simulink library "inp"  (R2021b)
settings: Solver=VariableStepAuto  StartTime=0.0  StopTime=10.0  RelTol=1e-3
undefined symbols (not defined in the file): C_TASK_5MS_S, FALSE, KINP_AcoreReadyToSlp_flg_ovrdflg, KINP_AcoreReadyToSlp_flg_ovrdval, KINP_AllowMovThd_OTA_enum_ovrdflg, KINP_AllowMovThd_OTA_enum_ovrdval, KINP_APSAngleTarget_Deg_ovrdflg, KINP_APSAngleTarget_Deg_ovrdval, KINP_APSDecReq_mps2_ovrdflg, KINP_APSDecReq_mps2_ovrdval, KINP_APSDecReqA_flg_ovrdflg, KINP_APSDecReqA_flg_ovrdval, KINP_APSDFLL_cm_ovrdflg, KINP_APSDFLL_cm_ovrdval, KINP_APSDFLR_cm_ovrdflg, KINP_APSDFLR_cm_ovrdval, KINP_APSDRLL_cm_ovrdflg, KINP_APSDRLL_cm_ovrdval, KINP_APSDRLR_cm_ovrdflg, KINP_APSDRLR_cm_ovrdval, KINP_APSExitCondition_enum_ovrdflg, KINP_APSExitCondition_enum_ovrdval, KINP_APSHWVer_enum_ovrdflg, KINP_APSHWVer_enum_ovrdval, KINP_APSProgressPCT_pct_ovrdflg, KINP_APSProgressPCT_pct_ovrdval, KINP_APSPwrReq_enum_ovrdflg, KINP_APSPwrReq_enum_ovrdval, KINP_APSReq_enum_ovrdflg, KINP_APSReq_enum_ovrdval, KINP_APSRQDisplay_enum_ovrdflg, KINP_APSRQDisplay_enum_ovrdval, KINP_APSRqEPASCtrl_flg_ovrdflg, KINP_APSRqEPASCtrl_flg_ovrdval, KINP_APSShiftPosnReq_enum_ovrdval, KINP_APSShiftPosnReq_enum_ovrflg, KINP_APSSpeedCMD_kph_ovrdval, KINP_APSSpeedCMD_kph_ovrflg, KINP_APSStaSystem_enum_ovrdflg, KINP_APSStaSystem_enum_ovrdval, KINP_APSSWVer_enum_ovrdflg, KINP_APSSWVer_enum_ovrdval, KINP_APSVMCReqA_flg_ovrdval, KINP_APSVMCReqA_flg_ovrflg, KINP_APSVRqEPASCtrl_flg_ovrdflg, KINP_APSVRqEPASCtrl_flg_ovrdval, KINP_AuxBattVolmV_mV_ovrdflg, KINP_AuxBattVolmV_mV_ovrdval, KINP_CAASSta_enum_ovrdflg, KINP_CAASSta_enum_ovrdval, KINP_CAASVMCReqA_flg_ovrdval, KINP_CAASVMCReqA_flg_ovrflg, KINP_CAN1BusOff_flg_ovrdflg, KINP_CAN1BusOff_flg_ovrdval, KINP_CAN2BusOff_flg_ovrdflg, KINP_CAN2BusOff_flg_ovrdval, KINP_CAN3BusOff_flg_ovrdflg, KINP_CAN3BusOff_flg_ovrdval, KINP_CAN4BusOff_flg_ovrdflg, KINP_CAN4BusOff_flg_ovrdval ... (+152)
libraries: FVT_lib x1037, hcu_lib x1
(part 33 of 34)

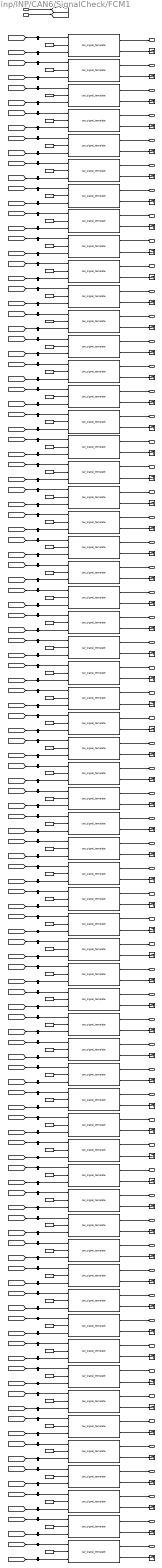
== system inp/INP/CAN6/SignalCheck/FCM1 ==
  BHAL_outputs : Inport
  inp_CanValid_bus : Inport  Port=2
  ACCComfortBandLower : FVT_lib/inp/can_signal_template  SystemSampleTime=-1  VariantActivationTime=update diagram  Latency=0  AutoFrameSizeCalculation=off
      link override defval: Value=KINP_ACCComfortBandLower_mps2_defval
      link override ovrdflg: Value=KINP_ACCComfortBandLower_mps2_ovrdflg
      link override ovrdval: Value=KINP_ACCComfortBandLower_mps2_ovrdval
  ACCComfortBandUpper : FVT_lib/inp/can_signal_template  SystemSampleTime=-1  VariantActivationTime=update diagram  Latency=0  AutoFrameSizeCalculation=off
      link override defval: Value=KINP_ACCComfortBandUpper_mps2_defval
      link override ovrdflg: Value=KINP_ACCComfortBandUpper_mps2_ovrdflg
      link override ovrdval: Value=KINP_ACCComfortBandUpper_mps2_ovrdval
  ACCJerkLowerLimit : FVT_lib/inp/can_signal_template  SystemSampleTime=-1  VariantActivationTime=update diagram  Latency=0  AutoFrameSizeCalculation=off
      link override defval: Value=KINP_ACCJerkLowerLimit_mps3_defval
      link override ovrdflg: Value=KINP_ACCJerkLowerLimit_mps3_ovrdflg
      link override ovrdval: Value=KINP_ACCJerkLowerLimit_mps3_ovrdval
  ACCJerkUpperLimit : FVT_lib/inp/can_signal_template  SystemSampleTime=-1  VariantActivationTime=update diagram  Latency=0  AutoFrameSizeCalculation=off
      link override defval: Value=KINP_ACCJerkUpperLimit_mps3_defval
      link override ovrdflg: Value=KINP_ACCJerkUpperLimit_mps3_ovrdflg
      link override ovrdval: Value=KINP_ACCJerkUpperLimit_mps3_ovrdval
  ACCObjDist : FVT_lib/inp/can_signal_template  SystemSampleTime=-1  VariantActivationTime=update diagram  Latency=0  AutoFrameSizeCalculation=off
      link override defval: Value=KINP_ACCObjDist_m_defval
      link override ovrdflg: Value=KINP_ACCObjDist_m_ovrdflg
      link override ovrdval: Value=KINP_ACCObjDist_m_ovrdval
  ACCObjDstLvl : FVT_lib/inp/can_signal_template  SystemSampleTime=-1  VariantActivationTime=update diagram  Latency=0  AutoFrameSizeCalculation=off
      link override defval: Value=KINP_ACCObjDstLvl_enum_defval
      link override ovrdflg: Value=KINP_ACCObjDstLvl_enum_ovrdflg
      link override ovrdval: Value=KINP_ACCObjDstLvl_enum_ovrdval
  ACCObjRelSpd : FVT_lib/inp/can_signal_template  SystemSampleTime=-1  VariantActivationTime=update diagram  Latency=0  AutoFrameSizeCalculation=off
      link override defval: Value=KINP_ACCObjRelSpd_mps_defval
      link override ovrdflg: Value=KINP_ACCObjRelSpd_mps_ovrdflg
      link override ovrdval: Value=KINP_ACCObjRelSpd_mps_ovrdval
  ACCRequiredAccel : FVT_lib/inp/can_signal_template  SystemSampleTime=-1  VariantActivationTime=update diagram  Latency=0  AutoFrameSizeCalculation=off
      link override defval: Value=KINP_ACCRequiredAccel_mps2_defval
      link override ovrdflg: Value=KINP_ACCRequiredAccel_mps2_ovrdflg
      link override ovrdval: Value=KINP_ACCRequiredAccel_mps2_ovrdval
  ACCTakeoverReq : FVT_lib/inp/can_signal_template  SystemSampleTime=-1  VariantActivationTime=update diagram  Latency=0  AutoFrameSizeCalculation=off
      link override defval: Value=KINP_ACCTakeoverReq_flg_defval
      link override ovrdflg: Value=KINP_ACCTakeoverReq_flg_ovrdflg
      link override ovrdval: Value=KINP_ACCTakeoverReq_flg_ovrdval
  ACCVehHoldReq : FVT_lib/inp/can_signal_template  SystemSampleTime=-1  VariantActivationTime=update diagram  Latency=0  AutoFrameSizeCalculation=off
      link override defval: Value=KINP_ACCVehHoldReq_flg_defval
      link override ovrdflg: Value=KINP_ACCVehHoldReq_flg_ovrdflg
      link override ovrdval: Value=KINP_ACCVehHoldReq_flg_ovrdval
  ADASACCSta : FVT_lib/inp/can_signal_template  SystemSampleTime=-1  VariantActivationTime=update diagram  Latency=0  AutoFrameSizeCalculation=off
      link override defval: Value=KINP_ADASACCSta_enum_defval
      link override ovrdflg: Value=KINP_ADASACCSta_enum_ovrdflg
      link override ovrdval: Value=KINP_ADASACCSta_enum_ovrdval
  ADASAEBReq : FVT_lib/inp/can_signal_template  SystemSampleTime=-1  VariantActivationTime=update diagram  Latency=0  AutoFrameSizeCalculation=off
      link override defval: Value=KINP_ADASAEBReq_enum_defval
      link override ovrdflg: Value=KINP_ADASAEBReq_enum_ovrdflg
      link override ovrdval: Value=KINP_ADASAEBReq_enum_ovrdval
  ADASAEBSta : FVT_lib/inp/can_signal_template  SystemSampleTime=-1  VariantActivationTime=update diagram  Latency=0  AutoFrameSizeCalculation=off
      link override defval: Value=KINP_ADASAEBSta_enum_defval
      link override ovrdflg: Value=KINP_ADASAEBSta_enum_ovrdflg
      link override ovrdval: Value=KINP_ADASAEBSta_enum_ovrdval
  ADASCAMSpdLim : FVT_lib/inp/can_signal_template  SystemSampleTime=-1  VariantActivationTime=update diagram  Latency=0  AutoFrameSizeCalculation=off
      link override defval: Value=KINP_ADASCAMSpdLim_enum_defval
      link override ovrdflg: Value=KINP_ADASCAMSpdLim_enum_ovrdflg
      link override ovrdval: Value=KINP_ADASCAMSpdLim_enum_ovrdval
  ADASDBSReq : FVT_lib/inp/can_signal_template  SystemSampleTime=-1  VariantActivationTime=update diagram  Latency=0  AutoFrameSizeCalculation=off
      link override defval: Value=KINP_ADASDBSReq_enum_defval
      link override ovrdflg: Value=KINP_ADASDBSReq_enum_ovrdflg
      link override ovrdval: Value=KINP_ADASDBSReq_enum_ovrdval
  ADASFCWMute : FVT_lib/inp/can_signal_template  SystemSampleTime=-1  VariantActivationTime=update diagram  Latency=0  AutoFrameSizeCalculation=off
      link override defval: Value=KINP_ADASFCWMute_flg_defval
      link override ovrdflg: Value=KINP_ADASFCWMute_flg_ovrdflg
      link override ovrdval: Value=KINP_ADASFCWMute_flg_ovrdval
  ADASFCWSta : FVT_lib/inp/can_signal_template  SystemSampleTime=-1  VariantActivationTime=update diagram  Latency=0  AutoFrameSizeCalculation=off
      link override defval: Value=KINP_ADASFCWSta_enum_defval
      link override ovrdflg: Value=KINP_ADASFCWSta_enum_ovrdflg
      link override ovrdval: Value=KINP_ADASFCWSta_enum_ovrdval
  ADASFaultSta : FVT_lib/inp/can_signal_template  SystemSampleTime=-1  VariantActivationTime=update diagram  Latency=0  AutoFrameSizeCalculation=off
      link override defval: Value=KINP_ADASFaultSta_flg_defval
      link override ovrdflg: Value=KINP_ADASFaultSta_flg_ovrdflg
      link override ovrdval: Value=KINP_ADASFaultSta_flg_ovrdval
  ADASFltWrnReq : FVT_lib/inp/can_signal_template  SystemSampleTime=-1  VariantActivationTime=update diagram  Latency=0  AutoFrameSizeCalculation=off
      link override defval: Value=KINP_ADASFltWrnReq_flg_defval
      link override ovrdflg: Value=KINP_ADASFltWrnReq_flg_ovrdflg
      link override ovrdval: Value=KINP_ADASFltWrnReq_flg_ovrdval
  ADASForceIdle : FVT_lib/inp/can_signal_template  SystemSampleTime=-1  VariantActivationTime=update diagram  Latency=0  AutoFrameSizeCalculation=off
      link override defval: Value=KINP_ADASForceIdle_flg_defval
      link override ovrdflg: Value=KINP_ADASForceIdle_flg_ovrdflg
      link override ovrdval: Value=KINP_ADASForceIdle_flg_ovrdval
  ADASISASta : FVT_lib/inp/can_signal_template  SystemSampleTime=-1  VariantActivationTime=update diagram  Latency=0  AutoFrameSizeCalculation=off
      link override defval: Value=KINP_ADASISASta_enum_defval
      link override ovrdflg: Value=KINP_ADASISASta_enum_ovrdflg
      link override ovrdval: Value=KINP_ADASISASta_enum_ovrdval
  ADASLDWMute : FVT_lib/inp/can_signal_template  SystemSampleTime=-1  VariantActivationTime=update diagram  Latency=0  AutoFrameSizeCalculation=off
      link override defval: Value=KINP_ADASLDWMute_flg_defval
      link override ovrdflg: Value=KINP_ADASLDWMute_flg_ovrdflg
      link override ovrdval: Value=KINP_ADASLDWMute_flg_ovrdval
  ADASLDWSta : FVT_lib/inp/can_signal_template  SystemSampleTime=-1  VariantActivationTime=update diagram  Latency=0  AutoFrameSizeCalculation=off
      link override defval: Value=KINP_ADASLDWSta_enum_defval
      link override ovrdflg: Value=KINP_ADASLDWSta_enum_ovrdflg
      link override ovrdval: Value=KINP_ADASLDWSta_enum_ovrdval
  ADASLFCHandsOffWarning : FVT_lib/inp/can_signal_template  SystemSampleTime=-1  VariantActivationTime=update diagram  Latency=0  AutoFrameSizeCalculation=off
      link override defval: Value=KINP_ADASLFCHandsOffWarning_enum_defval
      link override ovrdflg: Value=KINP_ADASLFCHandsOffWarning_enum_ovrdflg
      link override ovrdval: Value=KINP_ADASLFCHandsOffWarning_enum_ovrdval
  ADASLFCSta : FVT_lib/inp/can_signal_template  SystemSampleTime=-1  VariantActivationTime=update diagram  Latency=0  AutoFrameSizeCalculation=off
      link override defval: Value=KINP_ADASLFCSta_enum_defval
      link override ovrdflg: Value=KINP_ADASLFCSta_enum_ovrdflg
      link override ovrdval: Value=KINP_ADASLFCSta_enum_ovrdval
  ADASLFCWarnSound : FVT_lib/inp/can_signal_template  SystemSampleTime=-1  VariantActivationTime=update diagram  Latency=0  AutoFrameSizeCalculation=off
      link override defval: Value=KINP_ADASLFCWarnSound_enum_defval
      link override ovrdflg: Value=KINP_ADASLFCWarnSound_enum_ovrdflg
      link override ovrdval: Value=KINP_ADASLFCWarnSound_enum_ovrdval
  ADASLKASta : FVT_lib/inp/can_signal_template  SystemSampleTime=-1  VariantActivationTime=update diagram  Latency=0  AutoFrameSizeCalculation=off
      link override defval: Value=KINP_ADASLKASta_enum_defval
      link override ovrdflg: Value=KINP_ADASLKASta_enum_ovrdflg
      link override ovrdval: Value=KINP_ADASLKASta_enum_ovrdval
  ADASLaneModeL : FVT_lib/inp/can_signal_template  SystemSampleTime=-1  VariantActivationTime=update diagram  Latency=0  AutoFrameSizeCalculation=off
      link override defval: Value=KINP_ADASLaneModeL_enum_defval
      link override ovrdflg: Value=KINP_ADASLaneModeL_enum_ovrdflg
      link override ovrdval: Value=KINP_ADASLaneModeL_enum_ovrdval
  ADASLaneModeR : FVT_lib/inp/can_signal_template  SystemSampleTime=-1  VariantActivationTime=update diagram  Latency=0  AutoFrameSizeCalculation=off
      link override defval: Value=KINP_ADASLaneModeR_enum_defval
      link override ovrdflg: Value=KINP_ADASLaneModeR_enum_ovrdflg
      link override ovrdval: Value=KINP_ADASLaneModeR_enum_ovrdval
  ADASLanecurveL : FVT_lib/inp/can_signal_template  SystemSampleTime=-1  VariantActivationTime=update diagram  Latency=0  AutoFrameSizeCalculation=off
      link override defval: Value=KINP_ADASLanecurveL_raw32_defval
      link override ovrdflg: Value=KINP_ADASLanecurveL_raw32_ovrdflg
      link override ovrdval: Value=KINP_ADASLanecurveL_raw32_ovrdval
  ADASLanecurveR : FVT_lib/inp/can_signal_template  SystemSampleTime=-1  VariantActivationTime=update diagram  Latency=0  AutoFrameSizeCalculation=off
      link override defval: Value=KINP_ADASLanecurveR_raw32_defval
      link override ovrdflg: Value=KINP_ADASLanecurveR_raw32_ovrdflg
      link override ovrdval: Value=KINP_ADASLanecurveR_raw32_ovrdval
  ADASLanetypeL : FVT_lib/inp/can_signal_template  SystemSampleTime=-1  VariantActivationTime=update diagram  Latency=0  AutoFrameSizeCalculation=off
      link override defval: Value=KINP_ADASLanetypeL_enum_defval
      link override ovrdflg: Value=KINP_ADASLanetypeL_enum_ovrdflg
      link override ovrdval: Value=KINP_ADASLanetypeL_enum_ovrdval
  ADASLanetypeR : FVT_lib/inp/can_signal_template  SystemSampleTime=-1  VariantActivationTime=update diagram  Latency=0  AutoFrameSizeCalculation=off
      link override defval: Value=KINP_ADASLanetypeR_enum_defval
      link override ovrdflg: Value=KINP_ADASLanetypeR_enum_ovrdflg
      link override ovrdval: Value=KINP_ADASLanetypeR_enum_ovrdval
  ADASSLIFSpdLim : FVT_lib/inp/can_signal_template  SystemSampleTime=-1  VariantActivationTime=update diagram  Latency=0  AutoFrameSizeCalculation=off
      link override defval: Value=KINP_ADASSLIFSpdLim_enum_defval
      link override ovrdflg: Value=KINP_ADASSLIFSpdLim_enum_ovrdflg
      link override ovrdval: Value=KINP_ADASSLIFSpdLim_enum_ovrdval
  ADASSLIFSta : FVT_lib/inp/can_signal_template  SystemSampleTime=-1  VariantActivationTime=update diagram  Latency=0  AutoFrameSizeCalculation=off
      link override defval: Value=KINP_ADASSLIFSta_enum_defval
      link override ovrdflg: Value=KINP_ADASSLIFSta_enum_ovrdflg
      link override ovrdval: Value=KINP_ADASSLIFSta_enum_ovrdval
  ADASShftPosnReq : FVT_lib/inp/can_signal_template  SystemSampleTime=-1  VariantActivationTime=update diagram  Latency=0  AutoFrameSizeCalculation=off
      link override defval: Value=KINP_ADASShftPosnReq_enum_defval
      link override ovrdflg: Value=KINP_ADASShftPosnReq_enum_ovrdflg
      link override ovrdval: Value=KINP_ADASShftPosnReq_enum_ovrdval
  ADASShftPosnReqA : FVT_lib/inp/can_signal_template  SystemSampleTime=-1  VariantActivationTime=update diagram  Latency=0  AutoFrameSizeCalculation=off
      link override defval: Value=KINP_ADASShftPosnReqA_flg_defval
      link override ovrdflg: Value=KINP_ADASShftPosnReqA_flg_ovrdflg
      link override ovrdval: Value=KINP_ADASShftPosnReqA_flg_ovrdval
  ADASVehSpdLim : FVT_lib/inp/can_signal_template  SystemSampleTime=-1  VariantActivationTime=update diagram  Latency=0  AutoFrameSizeCalculation=off
      link override defval: Value=KINP_ADASVehSpdLim_enum_defval
      link override ovrdflg: Value=KINP_ADASVehSpdLim_enum_ovrdflg
      link override ovrdval: Value=KINP_ADASVehSpdLim_enum_ovrdval
  ADASWarningMsg : FVT_lib/inp/can_signal_template  SystemSampleTime=-1  VariantActivationTime=update diagram  Latency=0  AutoFrameSizeCalculation=off
      link override defval: Value=KINP_ADASWarningMsg_enum_defval
      link override ovrdflg: Value=KINP_ADASWarningMsg_enum_ovrdflg
      link override ovrdval: Value=KINP_ADASWarningMsg_enum_ovrdval
  AEBVehHoldReq : FVT_lib/inp/can_signal_template  SystemSampleTime=-1  VariantActivationTime=update diagram  Latency=0  AutoFrameSizeCalculation=off
      link override defval: Value=KINP_AEBVehHoldReq_flg_defval
      link override ovrdflg: Value=KINP_AEBVehHoldReq_flg_ovrdflg
      link override ovrdval: Value=KINP_AEBVehHoldReq_flg_ovrdval
  CameraBlockage : FVT_lib/inp/can_signal_template  SystemSampleTime=-1  VariantActivationTime=update diagram  Latency=0  AutoFrameSizeCalculation=off
      link override defval: Value=KINP_CameraBlockage_flg_defval
      link override ovrdflg: Value=KINP_CameraBlockage_flg_ovrdflg
      link override ovrdval: Value=KINP_CameraBlockage_flg_ovrdval
  FCM1Checksum : FVT_lib/inp/can_signal_template  SystemSampleTime=-1  VariantActivationTime=update diagram  Latency=0  AutoFrameSizeCalculation=off
      link override defval: Value=KINP_FCM1Checksum_enum_defval
      link override ovrdflg: Value=KINP_FCM1Checksum_enum_ovrdflg
      link override ovrdval: Value=KINP_FCM1Checksum_enum_ovrdval
  FCM1LifeCount : FVT_lib/inp/can_signal_template  SystemSampleTime=-1  VariantActivationTime=update diagram  Latency=0  AutoFrameSizeCalculation=off
      link override defval: Value=KINP_FCM1LifeCount_enum_defval
      link override ovrdflg: Value=KINP_FCM1LifeCount_enum_ovrdflg
      link override ovrdval: Value=KINP_FCM1LifeCount_enum_ovrdval
  FCMACCmode : FVT_lib/inp/can_signal_template  SystemSampleTime=-1  VariantActivationTime=update diagram  Latency=0  AutoFrameSizeCalculation=off
      link override defval: Value=KINP_FCMACCmode_enum_defval
      link override ovrdflg: Value=KINP_FCMACCmode_enum_ovrdflg
      link override ovrdval: Value=KINP_FCMACCmode_enum_ovrdval
  FCMLKAStrToqReq : FVT_lib/inp/can_signal_template  SystemSampleTime=-1  VariantActivationTime=update diagram  Latency=0  AutoFrameSizeCalculation=off
      link override defval: Value=KINP_FCMLKAStrToqReq_Nm_defval
      link override ovrdflg: Value=KINP_FCMLKAStrToqReq_Nm_ovrdflg
      link override ovrdval: Value=KINP_FCMLKAStrToqReq_Nm_ovrdval
  FCMLKATOIAct : FVT_lib/inp/can_signal_template  SystemSampleTime=-1  VariantActivationTime=update diagram  Latency=0  AutoFrameSizeCalculation=off
      link override defval: Value=KINP_FCMLKATOIAct_enum_defval
      link override ovrdflg: Value=KINP_FCMLKATOIAct_enum_ovrdflg
      link override ovrdval: Value=KINP_FCMLKATOIAct_enum_ovrdval
  FCMLKATOIFault : FVT_lib/inp/can_signal_template  SystemSampleTime=-1  VariantActivationTime=update diagram  Latency=0  AutoFrameSizeCalculation=off
      link override defval: Value=KINP_FCMLKATOIFault_flg_defval
      link override ovrdflg: Value=KINP_FCMLKATOIFault_flg_ovrdflg
      link override ovrdval: Value=KINP_FCMLKATOIFault_flg_ovrdval
  ForceLowBeam : FVT_lib/inp/can_signal_template  SystemSampleTime=-1  VariantActivationTime=update diagram  Latency=0  AutoFrameSizeCalculation=off
      link override defval: Value=KINP_ForceLowBeam_enum_defval
      link override ovrdflg: Value=KINP_ForceLowBeam_enum_ovrdflg
      link override ovrdval: Value=KINP_ForceLowBeam_enum_ovrdval
  HazardWarningReq : FVT_lib/inp/can_signal_template  SystemSampleTime=-1  VariantActivationTime=update diagram  Latency=0  AutoFrameSizeCalculation=off
      link override defval: Value=KINP_HazardWarningReq_flg_defval
      link override ovrdflg: Value=KINP_HazardWarningReq_flg_ovrdflg
      link override ovrdval: Value=KINP_HazardWarningReq_flg_ovrdval
  ISAWarningMsg : FVT_lib/inp/can_signal_template  SystemSampleTime=-1  VariantActivationTime=update diagram  Latency=0  AutoFrameSizeCalculation=off
      link override defval: Value=KINP_ISAWarningMsg_enum_defval
      link override ovrdflg: Value=KINP_ISAWarningMsg_enum_ovrdflg
      link override ovrdval: Value=KINP_ISAWarningMsg_enum_ovrdval
  LKAHODDisplayWarning : FVT_lib/inp/can_signal_template  SystemSampleTime=-1  VariantActivationTime=update diagram  Latency=0  AutoFrameSizeCalculation=off
      link override defval: Value=KINP_LKAHODDisplayWarning_flg_defval
      link override ovrdflg: Value=KINP_LKAHODDisplayWarning_flg_ovrdflg
      link override ovrdval: Value=KINP_LKAHODDisplayWarning_flg_ovrdval
  LKAHODSoundWarning : FVT_lib/inp/can_signal_template  SystemSampleTime=-1  VariantActivationTime=update diagram  Latency=0  AutoFrameSizeCalculation=off
      link override defval: Value=KINP_LKAHODSoundWarning_flg_defval
      link override ovrdflg: Value=KINP_LKAHODSoundWarning_flg_ovrdflg
      link override ovrdval: Value=KINP_LKAHODSoundWarning_flg_ovrdval
  LVDAACCStatusInformation : FVT_lib/inp/can_signal_template  SystemSampleTime=-1  VariantActivationTime=update diagram  Latency=0  AutoFrameSizeCalculation=off
      link override defval: Value=KINP_LVDAACCStatusInformation_flg_defval
      link override ovrdflg: Value=KINP_LVDAACCStatusInformation_flg_ovrdflg
      link override ovrdval: Value=KINP_LVDAACCStatusInformation_flg_ovrdval
  LVDADisabled : FVT_lib/inp/can_signal_template  SystemSampleTime=-1  VariantActivationTime=update diagram  Latency=0  AutoFrameSizeCalculation=off
      link override defval: Value=KINP_LVDADisabled_flg_defval
      link override ovrdflg: Value=KINP_LVDADisabled_flg_ovrdflg
      link override ovrdval: Value=KINP_LVDADisabled_flg_ovrdval
  LVDAFailinfo : FVT_lib/inp/can_signal_template  SystemSampleTime=-1  VariantActivationTime=update diagram  Latency=0  AutoFrameSizeCalculation=off
      link override defval: Value=KINP_LVDAFailinfo_flg_defval
      link override ovrdflg: Value=KINP_LVDAFailinfo_flg_ovrdflg
      link override ovrdval: Value=KINP_LVDAFailinfo_flg_ovrdval
  LVDAMuteSta : FVT_lib/inp/can_signal_template  SystemSampleTime=-1  VariantActivationTime=update diagram  Latency=0  AutoFrameSizeCalculation=off
      link override defval: Value=KINP_LVDAMuteSta_enum_defval
      link override ovrdflg: Value=KINP_LVDAMuteSta_enum_ovrdflg
      link override ovrdval: Value=KINP_LVDAMuteSta_enum_ovrdval
  LVDAWarning : FVT_lib/inp/can_signal_template  SystemSampleTime=-1  VariantActivationTime=update diagram  Latency=0  AutoFrameSizeCalculation=off
      link override defval: Value=KINP_LVDAWarning_flg_defval
      link override ovrdflg: Value=KINP_LVDAWarning_flg_ovrdflg
      link override ovrdval: Value=KINP_LVDAWarning_flg_ovrdval
  LeftTurnLightReq : FVT_lib/inp/can_signal_template  SystemSampleTime=-1  VariantActivationTime=update diagram  Latency=0  AutoFrameSizeCalculation=off
      link override defval: Value=KINP_LeftTurnLightReq_flg_defval
      link override ovrdflg: Value=KINP_LeftTurnLightReq_flg_ovrdflg
      link override ovrdval: Value=KINP_LeftTurnLightReq_flg_ovrdval
  RightTurnLightReq : FVT_lib/inp/can_signal_template  SystemSampleTime=-1  VariantActivationTime=update diagram  Latency=0  AutoFrameSizeCalculation=off
      link override defval: Value=KINP_RightTurnLightReq_flg_defval
      link override ovrdflg: Value=KINP_RightTurnLightReq_flg_ovrdflg
      link override ovrdval: Value=KINP_RightTurnLightReq_flg_ovrdval
  TargetType : FVT_lib/inp/can_signal_template  SystemSampleTime=-1  VariantActivationTime=update diagram  Latency=0  AutoFrameSizeCalculation=off
      link override defval: Value=KINP_TargetType_enum_defval
      link override ovrdflg: Value=KINP_TargetType_enum_ovrdflg
      link override ovrdval: Value=KINP_TargetType_enum_ovrdval
  Terminator_{1..61} (61 alike) : Terminator
  TimeGapLevel : FVT_lib/inp/can_signal_template  SystemSampleTime=-1  VariantActivationTime=update diagram  Latency=0  AutoFrameSizeCalculation=off
      link override defval: Value=KINP_TimeGapLevel_enum_defval
      link override ovrdflg: Value=KINP_TimeGapLevel_enum_ovrdflg
      link override ovrdval: Value=KINP_TimeGapLevel_enum_ovrdval
  True_VHAL_ACCComfortBandLower_mps2 : Constant  Value=TRUE  OutDataTypeStr=boolean
  True_VHAL_ACCComfortBandUpper_mps2 : Constant  Value=TRUE  OutDataTypeStr=boolean
  True_VHAL_ACCJerkLowerLimit_mps3 : Constant  Value=TRUE  OutDataTypeStr=boolean
  True_VHAL_ACCJerkUpperLimit_mps3 : Constant  Value=TRUE  OutDataTypeStr=boolean
  True_VHAL_ACCObjDist_m : Constant  Value=TRUE  OutDataTypeStr=boolean
  True_VHAL_ACCObjDstLvl_enum : Constant  Value=TRUE  OutDataTypeStr=boolean
  True_VHAL_ACCObjRelSpd_mps : Constant  Value=TRUE  OutDataTypeStr=boolean
  True_VHAL_ACCRequiredAccel_mps2 : Constant  Value=TRUE  OutDataTypeStr=boolean
  True_VHAL_ACCTakeoverReq_flg : Constant  Value=TRUE  OutDataTypeStr=boolean
  True_VHAL_ACCVehHoldReq_flg : Constant  Value=TRUE  OutDataTypeStr=boolean
  True_VHAL_ADASACCSta_enum : Constant  Value=TRUE  OutDataTypeStr=boolean
  True_VHAL_ADASAEBReq_enum : Constant  Value=TRUE  OutDataTypeStr=boolean
  True_VHAL_ADASAEBSta_enum : Constant  Value=TRUE  OutDataTypeStr=boolean
  True_VHAL_ADASCAMSpdLim_enum : Constant  Value=TRUE  OutDataTypeStr=boolean
  True_VHAL_ADASDBSReq_enum : Constant  Value=TRUE  OutDataTypeStr=boolean
  True_VHAL_ADASFCWMute_flg : Constant  Value=TRUE  OutDataTypeStr=boolean
  True_VHAL_ADASFCWSta_enum : Constant  Value=TRUE  OutDataTypeStr=boolean
  True_VHAL_ADASFaultSta_flg : Constant  Value=TRUE  OutDataTypeStr=boolean
  True_VHAL_ADASFltWrnReq_flg : Constant  Value=TRUE  OutDataTypeStr=boolean
  True_VHAL_ADASForceIdle_flg : Constant  Value=TRUE  OutDataTypeStr=boolean
  True_VHAL_ADASISASta_enum : Constant  Value=TRUE  OutDataTypeStr=boolean
  True_VHAL_ADASLDWMute_flg : Constant  Value=TRUE  OutDataTypeStr=boolean
  True_VHAL_ADASLDWSta_enum : Constant  Value=TRUE  OutDataTypeStr=boolean
  True_VHAL_ADASLFCHandsOffWarning_enum : Constant  Value=TRUE  OutDataTypeStr=boolean
  True_VHAL_ADASLFCSta_enum : Constant  Value=TRUE  OutDataTypeStr=boolean
  True_VHAL_ADASLFCWarnSound_enum : Constant  Value=TRUE  OutDataTypeStr=boolean
  True_VHAL_ADASLKASta_enum : Constant  Value=TRUE  OutDataTypeStr=boolean
  True_VHAL_ADASLaneModeL_enum : Constant  Value=TRUE  OutDataTypeStr=boolean
  True_VHAL_ADASLaneModeR_enum : Constant  Value=TRUE  OutDataTypeStr=boolean
  True_VHAL_ADASLanecurveL_raw32 : Constant  Value=TRUE  OutDataTypeStr=boolean
  True_VHAL_ADASLanecurveR_raw32 : Constant  Value=TRUE  OutDataTypeStr=boolean
  True_VHAL_ADASLanetypeL_enum : Constant  Value=TRUE  OutDataTypeStr=boolean
  True_VHAL_ADASLanetypeR_enum : Constant  Value=TRUE  OutDataTypeStr=boolean
  True_VHAL_ADASSLIFSpdLim_enum : Constant  Value=TRUE  OutDataTypeStr=boolean
  True_VHAL_ADASSLIFSta_enum : Constant  Value=TRUE  OutDataTypeStr=boolean
  True_VHAL_ADASShftPosnReqA_flg : Constant  Value=TRUE  OutDataTypeStr=boolean
  True_VHAL_ADASShftPosnReq_enum : Constant  Value=TRUE  OutDataTypeStr=boolean
  True_VHAL_ADASVehSpdLim_enum : Constant  Value=TRUE  OutDataTypeStr=boolean
  True_VHAL_ADASWarningMsg_enum : Constant  Value=TRUE  OutDataTypeStr=boolean
  True_VHAL_AEBVehHoldReq_flg : Constant  Value=TRUE  OutDataTypeStr=boolean
  True_VHAL_CameraBlockage_flg : Constant  Value=TRUE  OutDataTypeStr=boolean
  True_VHAL_FCM1Checksum_enum : Constant  Value=TRUE  OutDataTypeStr=boolean
  True_VHAL_FCM1LifeCount_enum : Constant  Value=TRUE  OutDataTypeStr=boolean
  True_VHAL_FCMACCmode_enum : Constant  Value=TRUE  OutDataTypeStr=boolean
  True_VHAL_FCMLKAStrToqReq_Nm : Constant  Value=TRUE  OutDataTypeStr=boolean
  True_VHAL_FCMLKATOIAct_enum : Constant  Value=TRUE  OutDataTypeStr=boolean
  True_VHAL_FCMLKATOIFault_flg : Constant  Value=TRUE  OutDataTypeStr=boolean
  True_VHAL_ForceLowBeam_enum : Constant  Value=TRUE  OutDataTypeStr=boolean
  True_VHAL_HazardWarningReq_flg : Constant  Value=TRUE  OutDataTypeStr=boolean
  True_VHAL_ISAWarningMsg_enum : Constant  Value=TRUE  OutDataTypeStr=boolean
  True_VHAL_LKAHODDisplayWarning_flg : Constant  Value=TRUE  OutDataTypeStr=boolean
  True_VHAL_LKAHODSoundWarning_flg : Constant  Value=TRUE  OutDataTypeStr=boolean
  True_VHAL_LVDAACCStatusInformation_flg : Constant  Value=TRUE  OutDataTypeStr=boolean
  True_VHAL_LVDADisabled_flg : Constant  Value=TRUE  OutDataTypeStr=boolean
  True_VHAL_LVDAFailinfo_flg : Constant  Value=TRUE  OutDataTypeStr=boolean
  True_VHAL_LVDAMuteSta_enum : Constant  Value=TRUE  OutDataTypeStr=boolean
  True_VHAL_LVDAWarning_flg : Constant  Value=TRUE  OutDataTypeStr=boolean
  True_VHAL_LeftTurnLightReq_flg : Constant  Value=TRUE  OutDataTypeStr=boolean
  True_VHAL_RightTurnLightReq_flg : Constant  Value=TRUE  OutDataTypeStr=boolean
  True_VHAL_TargetType_enum : Constant  Value=TRUE  OutDataTypeStr=boolean
  True_VHAL_TimeGapLevel_enum : Constant  Value=TRUE  OutDataTypeStr=boolean
  slr1_{1..61} (61 alike) : BusSelector  OutputSignals=VINP_CANMsgValidFCM1_flg
  slr_VHAL_ACCComfortBandLower_mps2 : BusSelector  OutputSignals=VHAL_ACCComfortBandLower_mps2
  slr_VHAL_ACCComfortBandUpper_mps2 : BusSelector  OutputSignals=VHAL_ACCComfortBandUpper_mps2
  slr_VHAL_ACCJerkLowerLimit_mps3 : BusSelector  OutputSignals=VHAL_ACCJerkLowerLimit_mps3
  slr_VHAL_ACCJerkUpperLimit_mps3 : BusSelector  OutputSignals=VHAL_ACCJerkUpperLimit_mps3
  slr_VHAL_ACCObjDist_m : BusSelector  OutputSignals=VHAL_ACCObjDist_m
  slr_VHAL_ACCObjDstLvl_enum : BusSelector  OutputSignals=VHAL_ACCObjDstLvl_enum
  slr_VHAL_ACCObjRelSpd_mps : BusSelector  OutputSignals=VHAL_ACCObjRelSpd_mps
  slr_VHAL_ACCRequiredAccel_mps2 : BusSelector  OutputSignals=VHAL_ACCRequiredAccel_mps2
  slr_VHAL_ACCTakeoverReq_flg : BusSelector  OutputSignals=VHAL_ACCTakeoverReq_flg
  slr_VHAL_ACCVehHoldReq_flg : BusSelector  OutputSignals=VHAL_ACCVehHoldReq_flg
  slr_VHAL_ADASACCSta_enum : BusSelector  OutputSignals=VHAL_ADASACCSta_enum
  slr_VHAL_ADASAEBReq_enum : BusSelector  OutputSignals=VHAL_ADASAEBReq_enum
  slr_VHAL_ADASAEBSta_enum : BusSelector  OutputSignals=VHAL_ADASAEBSta_enum
  slr_VHAL_ADASCAMSpdLim_enum : BusSelector  OutputSignals=VHAL_ADASCAMSpdLim_enum
  slr_VHAL_ADASDBSReq_enum : BusSelector  OutputSignals=VHAL_ADASDBSReq_enum
  slr_VHAL_ADASFCWMute_flg : BusSelector  OutputSignals=VHAL_ADASFCWMute_flg
  slr_VHAL_ADASFCWSta_enum : BusSelector  OutputSignals=VHAL_ADASFCWSta_enum
  slr_VHAL_ADASFaultSta_flg : BusSelector  OutputSignals=VHAL_ADASFaultSta_flg
  slr_VHAL_ADASFltWrnReq_flg : BusSelector  OutputSignals=VHAL_ADASFltWrnReq_flg
  slr_VHAL_ADASForceIdle_flg : BusSelector  OutputSignals=VHAL_ADASForceIdle_flg
  slr_VHAL_ADASISASta_enum : BusSelector  OutputSignals=VHAL_ADASISASta_enum
  slr_VHAL_ADASLDWMute_flg : BusSelector  OutputSignals=VHAL_ADASLDWMute_flg
  slr_VHAL_ADASLDWSta_enum : BusSelector  OutputSignals=VHAL_ADASLDWSta_enum
  slr_VHAL_ADASLFCHandsOffWarning_enum : BusSelector  OutputSignals=VHAL_ADASLFCHandsOffWarning_enum
  slr_VHAL_ADASLFCSta_enum : BusSelector  OutputSignals=VHAL_ADASLFCSta_enum
  slr_VHAL_ADASLFCWarnSound_enum : BusSelector  OutputSignals=VHAL_ADASLFCWarnSound_enum
  slr_VHAL_ADASLKASta_enum : BusSelector  OutputSignals=VHAL_ADASLKASta_enum
  slr_VHAL_ADASLaneModeL_enum : BusSelector  OutputSignals=VHAL_ADASLaneModeL_enum
  slr_VHAL_ADASLaneModeR_enum : BusSelector  OutputSignals=VHAL_ADASLaneModeR_enum
  slr_VHAL_ADASLanecurveL_raw32 : BusSelector  OutputSignals=VHAL_ADASLanecurveL_raw32
  slr_VHAL_ADASLanecurveR_raw32 : BusSelector  OutputSignals=VHAL_ADASLanecurveR_raw32
  slr_VHAL_ADASLanetypeL_enum : BusSelector  OutputSignals=VHAL_ADASLanetypeL_enum
  slr_VHAL_ADASLanetypeR_enum : BusSelector  OutputSignals=VHAL_ADASLanetypeR_enum
  slr_VHAL_ADASSLIFSpdLim_enum : BusSelector  OutputSignals=VHAL_ADASSLIFSpdLim_enum
  slr_VHAL_ADASSLIFSta_enum : BusSelector  OutputSignals=VHAL_ADASSLIFSta_enum
  slr_VHAL_ADASShftPosnReqA_flg : BusSelector  OutputSignals=VHAL_ADASShftPosnReqA_flg
  slr_VHAL_ADASShftPosnReq_enum : BusSelector  OutputSignals=VHAL_ADASShftPosnReq_enum
  slr_VHAL_ADASVehSpdLim_enum : BusSelector  OutputSignals=VHAL_ADASVehSpdLim_enum
  slr_VHAL_ADASWarningMsg_enum : BusSelector  OutputSignals=VHAL_ADASWarningMsg_enum
  slr_VHAL_AEBVehHoldReq_flg : BusSelector  OutputSignals=VHAL_AEBVehHoldReq_flg
  slr_VHAL_CameraBlockage_flg : BusSelector  OutputSignals=VHAL_CameraBlockage_flg
  slr_VHAL_FCM1Checksum_enum : BusSelector  OutputSignals=VHAL_FCM1Checksum_enum
  slr_VHAL_FCM1LifeCount_enum : BusSelector  OutputSignals=VHAL_FCM1LifeCount_enum
  slr_VHAL_FCMACCmode_enum : BusSelector  OutputSignals=VHAL_FCMACCmode_enum
  slr_VHAL_FCMLKAStrToqReq_Nm : BusSelector  OutputSignals=VHAL_FCMLKAStrToqReq_Nm
  slr_VHAL_FCMLKATOIAct_enum : BusSelector  OutputSignals=VHAL_FCMLKATOIAct_enum
  slr_VHAL_FCMLKATOIFault_flg : BusSelector  OutputSignals=VHAL_FCMLKATOIFault_flg
  slr_VHAL_ForceLowBeam_enum : BusSelector  OutputSignals=VHAL_ForceLowBeam_enum
  slr_VHAL_HazardWarningReq_flg : BusSelector  OutputSignals=VHAL_HazardWarningReq_flg
  slr_VHAL_ISAWarningMsg_enum : BusSelector  OutputSignals=VHAL_ISAWarningMsg_enum
  slr_VHAL_LKAHODDisplayWarning_flg : BusSelector  OutputSignals=VHAL_LKAHODDisplayWarning_flg
  slr_VHAL_LKAHODSoundWarning_flg : BusSelector  OutputSignals=VHAL_LKAHODSoundWarning_flg
  slr_VHAL_LVDAACCStatusInformation_flg : BusSelector  OutputSignals=VHAL_LVDAACCStatusInformation_flg
  slr_VHAL_LVDADisabled_flg : BusSelector  OutputSignals=VHAL_LVDADisabled_flg
  slr_VHAL_LVDAFailinfo_flg : BusSelector  OutputSignals=VHAL_LVDAFailinfo_flg
  slr_VHAL_LVDAMuteSta_enum : BusSelector  OutputSignals=VHAL_LVDAMuteSta_enum
  slr_VHAL_LVDAWarning_flg : BusSelector  OutputSignals=VHAL_LVDAWarning_flg
  slr_VHAL_LeftTurnLightReq_flg : BusSelector  OutputSignals=VHAL_LeftTurnLightReq_flg
  slr_VHAL_RightTurnLightReq_flg : BusSelector  OutputSignals=VHAL_RightTurnLightReq_flg
  slr_VHAL_TargetType_enum : BusSelector  OutputSignals=VHAL_TargetType_enum
  slr_VHAL_TimeGapLevel_enum : BusSelector  OutputSignals=VHAL_TimeGapLevel_enum
  VINP_ACCComfortBandLower_mps2 : Outport
  VINP_ACCComfortBandUpper_mps2 : Outport  Port=2
  VINP_ACCJerkLowerLimit_mps3 : Outport  Port=3
  VINP_ACCJerkUpperLimit_mps3 : Outport  Port=4
  VINP_ACCObjDist_m : Outport  Port=5
  VINP_ACCObjDstLvl_enum : Outport  Port=6
  VINP_ACCObjRelSpd_mps : Outport  Port=7
  VINP_ACCRequiredAccel_mps2 : Outport  Port=8
  VINP_ACCTakeoverReq_flg : Outport  Port=9
  VINP_ACCVehHoldReq_flg : Outport  Port=10
  VINP_ADASACCSta_enum : Outport  Port=11
  VINP_ADASAEBReq_enum : Outport  Port=12
  VINP_ADASAEBSta_enum : Outport  Port=13
  VINP_ADASCAMSpdLim_enum : Outport  Port=14
  VINP_ADASDBSReq_enum : Outport  Port=15
  VINP_ADASFCWMute_flg : Outport  Port=16
  VINP_ADASFCWSta_enum : Outport  Port=17
  VINP_ADASFaultSta_flg : Outport  Port=18
  VINP_ADASFltWrnReq_flg : Outport  Port=19
  VINP_ADASForceIdle_flg : Outport  Port=20
  VINP_ADASISASta_enum : Outport  Port=21
  VINP_ADASLDWMute_flg : Outport  Port=22
  VINP_ADASLDWSta_enum : Outport  Port=23
  VINP_ADASLFCHandsOffWarning_enum : Outport  Port=24
  VINP_ADASLFCSta_enum : Outport  Port=25
  VINP_ADASLFCWarnSound_enum : Outport  Port=26
  VINP_ADASLKASta_enum : Outport  Port=27
  VINP_ADASLaneModeL_enum : Outport  Port=28
  VINP_ADASLaneModeR_enum : Outport  Port=29
  VINP_ADASLanecurveL_raw32 : Outport  Port=30
  VINP_ADASLanecurveR_raw32 : Outport  Port=31
  VINP_ADASLanetypeL_enum : Outport  Port=32
  VINP_ADASLanetypeR_enum : Outport  Port=33
  VINP_ADASSLIFSpdLim_enum : Outport  Port=34
  VINP_ADASSLIFSta_enum : Outport  Port=35
  VINP_ADASShftPosnReq_enum : Outport  Port=36
  VINP_ADASShftPosnReqA_flg : Outport  Port=37
  VINP_ADASVehSpdLim_enum : Outport  Port=38
  VINP_ADASWarningMsg_enum : Outport  Port=39
  VINP_AEBVehHoldReq_flg : Outport  Port=40
  VINP_CameraBlockage_flg : Outport  Port=41
  VINP_FCM1Checksum_enum : Outport  Port=42
  VINP_FCM1LifeCount_enum : Outport  Port=43
  VINP_FCMACCmode_enum : Outport  Port=44
  VINP_FCMLKAStrToqReq_Nm : Outport  Port=45
  VINP_FCMLKATOIAct_enum : Outport  Port=46
  VINP_FCMLKATOIFault_flg : Outport  Port=47
  VINP_ForceLowBeam_enum : Outport  Port=48
  VINP_HazardWarningReq_flg : Outport  Port=49
  VINP_ISAWarningMsg_enum : Outport  Port=50
  VINP_LKAHODDisplayWarning_flg : Outport  Port=51
  VINP_LKAHODSoundWarning_flg : Outport  Port=52
  VINP_LVDAACCStatusInformation_flg : Outport  Port=53
  VINP_LVDADisabled_flg : Outport  Port=54
  VINP_LVDAFailinfo_flg : Outport  Port=55
  VINP_LVDAMuteSta_enum : Outport  Port=56
  VINP_LVDAWarning_flg : Outport  Port=57
  VINP_LeftTurnLightReq_flg : Outport  Port=58
  VINP_RightTurnLightReq_flg : Outport  Port=59
  VINP_TargetType_enum : Outport  Port=60
  VINP_TimeGapLevel_enum : Outport  Port=61
  wires:
  BHAL_outputs/1 -> [BHAL_outputs]
  inp_CanValid_bus/1 -> [inp_CanValid_bus]
  [BHAL_outputs] -> slr_VHAL_ACCComfortBandLower_mps2/1
  slr_VHAL_ACCComfortBandLower_mps2/1 -> ACCComfortBandLower/1  "<VHAL_ACCComfortBandLower_mps2>"
  True_VHAL_ACCComfortBandLower_mps2/1 -> ACCComfortBandLower/2
  [inp_CanValid_bus] -> slr1_1/1
  slr1_1/1 -> ACCComfortBandLower/3  "<VINP_CANMsgValidFCM1_flg>"
  ACCComfortBandLower/1 -> VINP_ACCComfortBandLower_mps2/1  "VINP_ACCComfortBandLower_mps2"
  ACCComfortBandLower/2 -> Terminator_1/1
  [BHAL_outputs] -> slr_VHAL_ACCComfortBandUpper_mps2/1
  slr_VHAL_ACCComfortBandUpper_mps2/1 -> ACCComfortBandUpper/1  "<VHAL_ACCComfortBandUpper_mps2>"
  True_VHAL_ACCComfortBandUpper_mps2/1 -> ACCComfortBandUpper/2
  [inp_CanValid_bus] -> slr1_2/1
  slr1_2/1 -> ACCComfortBandUpper/3  "<VINP_CANMsgValidFCM1_flg>"
  ACCComfortBandUpper/1 -> VINP_ACCComfortBandUpper_mps2/1  "VINP_ACCComfortBandUpper_mps2"
  ACCComfortBandUpper/2 -> Terminator_2/1
  [BHAL_outputs] -> slr_VHAL_ACCJerkLowerLimit_mps3/1
  slr_VHAL_ACCJerkLowerLimit_mps3/1 -> ACCJerkLowerLimit/1  "<VHAL_ACCJerkLowerLimit_mps3>"
  True_VHAL_ACCJerkLowerLimit_mps3/1 -> ACCJerkLowerLimit/2
  [inp_CanValid_bus] -> slr1_3/1
  slr1_3/1 -> ACCJerkLowerLimit/3  "<VINP_CANMsgValidFCM1_flg>"
  ACCJerkLowerLimit/1 -> VINP_ACCJerkLowerLimit_mps3/1  "VINP_ACCJerkLowerLimit_mps3"
  ACCJerkLowerLimit/2 -> Terminator_3/1
  [BHAL_outputs] -> slr_VHAL_ACCJerkUpperLimit_mps3/1
  slr_VHAL_ACCJerkUpperLimit_mps3/1 -> ACCJerkUpperLimit/1  "<VHAL_ACCJerkUpperLimit_mps3>"
  True_VHAL_ACCJerkUpperLimit_mps3/1 -> ACCJerkUpperLimit/2
  [inp_CanValid_bus] -> slr1_4/1
  slr1_4/1 -> ACCJerkUpperLimit/3  "<VINP_CANMsgValidFCM1_flg>"
  ACCJerkUpperLimit/1 -> VINP_ACCJerkUpperLimit_mps3/1  "VINP_ACCJerkUpperLimit_mps3"
  ACCJerkUpperLimit/2 -> Terminator_4/1
  [BHAL_outputs] -> slr_VHAL_ACCObjDist_m/1
  slr_VHAL_ACCObjDist_m/1 -> ACCObjDist/1  "<VHAL_ACCObjDist_m>"
  True_VHAL_ACCObjDist_m/1 -> ACCObjDist/2
  [inp_CanValid_bus] -> slr1_5/1
  slr1_5/1 -> ACCObjDist/3  "<VINP_CANMsgValidFCM1_flg>"
  ACCObjDist/1 -> VINP_ACCObjDist_m/1  "VINP_ACCObjDist_m"
  ACCObjDist/2 -> Terminator_5/1
  [BHAL_outputs] -> slr_VHAL_ACCObjDstLvl_enum/1
  slr_VHAL_ACCObjDstLvl_enum/1 -> ACCObjDstLvl/1  "<VHAL_ACCObjDstLvl_enum>"
  True_VHAL_ACCObjDstLvl_enum/1 -> ACCObjDstLvl/2
  [inp_CanValid_bus] -> slr1_6/1
  slr1_6/1 -> ACCObjDstLvl/3  "<VINP_CANMsgValidFCM1_flg>"
  ACCObjDstLvl/1 -> VINP_ACCObjDstLvl_enum/1  "VINP_ACCObjDstLvl_enum"
  ACCObjDstLvl/2 -> Terminator_6/1
  [BHAL_outputs] -> slr_VHAL_ACCObjRelSpd_mps/1
  slr_VHAL_ACCObjRelSpd_mps/1 -> ACCObjRelSpd/1  "<VHAL_ACCObjRelSpd_mps>"
  True_VHAL_ACCObjRelSpd_mps/1 -> ACCObjRelSpd/2
  [inp_CanValid_bus] -> slr1_7/1
  slr1_7/1 -> ACCObjRelSpd/3  "<VINP_CANMsgValidFCM1_flg>"
  ACCObjRelSpd/1 -> VINP_ACCObjRelSpd_mps/1  "VINP_ACCObjRelSpd_mps"
  ACCObjRelSpd/2 -> Terminator_7/1
  [BHAL_outputs] -> slr_VHAL_ACCRequiredAccel_mps2/1
  slr_VHAL_ACCRequiredAccel_mps2/1 -> ACCRequiredAccel/1  "<VHAL_ACCRequiredAccel_mps2>"
  True_VHAL_ACCRequiredAccel_mps2/1 -> ACCRequiredAccel/2
  [inp_CanValid_bus] -> slr1_8/1
  slr1_8/1 -> ACCRequiredAccel/3  "<VINP_CANMsgValidFCM1_flg>"
  ACCRequiredAccel/1 -> VINP_ACCRequiredAccel_mps2/1  "VINP_ACCRequiredAccel_mps2"
  ACCRequiredAccel/2 -> Terminator_8/1
  [BHAL_outputs] -> slr_VHAL_ACCTakeoverReq_flg/1
  slr_VHAL_ACCTakeoverReq_flg/1 -> ACCTakeoverReq/1  "<VHAL_ACCTakeoverReq_flg>"
  True_VHAL_ACCTakeoverReq_flg/1 -> ACCTakeoverReq/2
  [inp_CanValid_bus] -> slr1_9/1
  slr1_9/1 -> ACCTakeoverReq/3  "<VINP_CANMsgValidFCM1_flg>"
  ACCTakeoverReq/1 -> VINP_ACCTakeoverReq_flg/1  "VINP_ACCTakeoverReq_flg"
  ACCTakeoverReq/2 -> Terminator_9/1
  [BHAL_outputs] -> slr_VHAL_ACCVehHoldReq_flg/1
  slr_VHAL_ACCVehHoldReq_flg/1 -> ACCVehHoldReq/1  "<VHAL_ACCVehHoldReq_flg>"
  True_VHAL_ACCVehHoldReq_flg/1 -> ACCVehHoldReq/2
  [inp_CanValid_bus] -> slr1_10/1
  slr1_10/1 -> ACCVehHoldReq/3  "<VINP_CANMsgValidFCM1_flg>"
  ACCVehHoldReq/1 -> VINP_ACCVehHoldReq_flg/1  "VINP_ACCVehHoldReq_flg"
  ACCVehHoldReq/2 -> Terminator_10/1
  [BHAL_outputs] -> slr_VHAL_ADASACCSta_enum/1
  slr_VHAL_ADASACCSta_enum/1 -> ADASACCSta/1  "<VHAL_ADASACCSta_enum>"
  True_VHAL_ADASACCSta_enum/1 -> ADASACCSta/2
  [inp_CanValid_bus] -> slr1_11/1
  slr1_11/1 -> ADASACCSta/3  "<VINP_CANMsgValidFCM1_flg>"
  ADASACCSta/1 -> VINP_ADASACCSta_enum/1  "VINP_ADASACCSta_enum"
  ADASACCSta/2 -> Terminator_11/1
  [BHAL_outputs] -> slr_VHAL_ADASAEBReq_enum/1
  slr_VHAL_ADASAEBReq_enum/1 -> ADASAEBReq/1  "<VHAL_ADASAEBReq_enum>"
  True_VHAL_ADASAEBReq_enum/1 -> ADASAEBReq/2
  [inp_CanValid_bus] -> slr1_12/1
  slr1_12/1 -> ADASAEBReq/3  "<VINP_CANMsgValidFCM1_flg>"
  ADASAEBReq/1 -> VINP_ADASAEBReq_enum/1  "VINP_ADASAEBReq_enum"
  ADASAEBReq/2 -> Terminator_12/1
  [BHAL_outputs] -> slr_VHAL_ADASAEBSta_enum/1
  slr_VHAL_ADASAEBSta_enum/1 -> ADASAEBSta/1  "<VHAL_ADASAEBSta_enum>"
  True_VHAL_ADASAEBSta_enum/1 -> ADASAEBSta/2
  [inp_CanValid_bus] -> slr1_13/1
  slr1_13/1 -> ADASAEBSta/3  "<VINP_CANMsgValidFCM1_flg>"
  ADASAEBSta/1 -> VINP_ADASAEBSta_enum/1  "VINP_ADASAEBSta_enum"
  ADASAEBSta/2 -> Terminator_13/1
  [BHAL_outputs] -> slr_VHAL_ADASCAMSpdLim_enum/1
  slr_VHAL_ADASCAMSpdLim_enum/1 -> ADASCAMSpdLim/1  "<VHAL_ADASCAMSpdLim_enum>"
  True_VHAL_ADASCAMSpdLim_enum/1 -> ADASCAMSpdLim/2
  [inp_CanValid_bus] -> slr1_14/1
  slr1_14/1 -> ADASCAMSpdLim/3  "<VINP_CANMsgValidFCM1_flg>"
  ADASCAMSpdLim/1 -> VINP_ADASCAMSpdLim_enum/1  "VINP_ADASCAMSpdLim_enum"
  ADASCAMSpdLim/2 -> Terminator_14/1
  [BHAL_outputs] -> slr_VHAL_ADASDBSReq_enum/1
  slr_VHAL_ADASDBSReq_enum/1 -> ADASDBSReq/1  "<VHAL_ADASDBSReq_enum>"
  True_VHAL_ADASDBSReq_enum/1 -> ADASDBSReq/2
  [inp_CanValid_bus] -> slr1_15/1
  slr1_15/1 -> ADASDBSReq/3  "<VINP_CANMsgValidFCM1_flg>"
  ADASDBSReq/1 -> VINP_ADASDBSReq_enum/1  "VINP_ADASDBSReq_enum"
  ADASDBSReq/2 -> Terminator_15/1
  [BHAL_outputs] -> slr_VHAL_ADASFCWMute_flg/1
  slr_VHAL_ADASFCWMute_flg/1 -> ADASFCWMute/1  "<VHAL_ADASFCWMute_flg>"
  True_VHAL_ADASFCWMute_flg/1 -> ADASFCWMute/2
  [inp_CanValid_bus] -> slr1_16/1
  slr1_16/1 -> ADASFCWMute/3  "<VINP_CANMsgValidFCM1_flg>"
  ADASFCWMute/1 -> VINP_ADASFCWMute_flg/1  "VINP_ADASFCWMute_flg"
  ADASFCWMute/2 -> Terminator_16/1
  [BHAL_outputs] -> slr_VHAL_ADASFCWSta_enum/1
  slr_VHAL_ADASFCWSta_enum/1 -> ADASFCWSta/1  "<VHAL_ADASFCWSta_enum>"
  True_VHAL_ADASFCWSta_enum/1 -> ADASFCWSta/2
  [inp_CanValid_bus] -> slr1_17/1
  slr1_17/1 -> ADASFCWSta/3  "<VINP_CANMsgValidFCM1_flg>"
  ADASFCWSta/1 -> VINP_ADASFCWSta_enum/1  "VINP_ADASFCWSta_enum"
  ADASFCWSta/2 -> Terminator_17/1
  [BHAL_outputs] -> slr_VHAL_ADASFaultSta_flg/1
  slr_VHAL_ADASFaultSta_flg/1 -> ADASFaultSta/1  "<VHAL_ADASFaultSta_flg>"
  True_VHAL_ADASFaultSta_flg/1 -> ADASFaultSta/2
  [inp_CanValid_bus] -> slr1_18/1
  slr1_18/1 -> ADASFaultSta/3  "<VINP_CANMsgValidFCM1_flg>"
  ADASFaultSta/1 -> VINP_ADASFaultSta_flg/1  "VINP_ADASFaultSta_flg"
  ADASFaultSta/2 -> Terminator_18/1
  [BHAL_outputs] -> slr_VHAL_ADASFltWrnReq_flg/1
  slr_VHAL_ADASFltWrnReq_flg/1 -> ADASFltWrnReq/1  "<VHAL_ADASFltWrnReq_flg>"
  True_VHAL_ADASFltWrnReq_flg/1 -> ADASFltWrnReq/2
  [inp_CanValid_bus] -> slr1_19/1
  slr1_19/1 -> ADASFltWrnReq/3  "<VINP_CANMsgValidFCM1_flg>"
  ADASFltWrnReq/1 -> VINP_ADASFltWrnReq_flg/1  "VINP_ADASFltWrnReq_flg"
  ADASFltWrnReq/2 -> Terminator_19/1
  [BHAL_outputs] -> slr_VHAL_ADASForceIdle_flg/1
  slr_VHAL_ADASForceIdle_flg/1 -> ADASForceIdle/1  "<VHAL_ADASForceIdle_flg>"
  True_VHAL_ADASForceIdle_flg/1 -> ADASForceIdle/2
  [inp_CanValid_bus] -> slr1_20/1
  slr1_20/1 -> ADASForceIdle/3  "<VINP_CANMsgValidFCM1_flg>"
  ADASForceIdle/1 -> VINP_ADASForceIdle_flg/1  "VINP_ADASForceIdle_flg"
  ADASForceIdle/2 -> Terminator_20/1
  [BHAL_outputs] -> slr_VHAL_ADASISASta_enum/1
  slr_VHAL_ADASISASta_enum/1 -> ADASISASta/1  "<VHAL_ADASISASta_enum>"
  True_VHAL_ADASISASta_enum/1 -> ADASISASta/2
  [inp_CanValid_bus] -> slr1_21/1
  slr1_21/1 -> ADASISASta/3  "<VINP_CANMsgValidFCM1_flg>"
  ADASISASta/1 -> VINP_ADASISASta_enum/1  "VINP_ADASISASta_enum"
  ADASISASta/2 -> Terminator_21/1
  [BHAL_outputs] -> slr_VHAL_ADASLDWMute_flg/1
  slr_VHAL_ADASLDWMute_flg/1 -> ADASLDWMute/1  "<VHAL_ADASLDWMute_flg>"
  True_VHAL_ADASLDWMute_flg/1 -> ADASLDWMute/2
  [inp_CanValid_bus] -> slr1_22/1
  slr1_22/1 -> ADASLDWMute/3  "<VINP_CANMsgValidFCM1_flg>"
  ADASLDWMute/1 -> VINP_ADASLDWMute_flg/1  "VINP_ADASLDWMute_flg"
  ADASLDWMute/2 -> Terminator_22/1
  [BHAL_outputs] -> slr_VHAL_ADASLDWSta_enum/1
  slr_VHAL_ADASLDWSta_enum/1 -> ADASLDWSta/1  "<VHAL_ADASLDWSta_enum>"
  True_VHAL_ADASLDWSta_enum/1 -> ADASLDWSta/2
  [inp_CanValid_bus] -> slr1_23/1
  slr1_23/1 -> ADASLDWSta/3  "<VINP_CANMsgValidFCM1_flg>"
  ADASLDWSta/1 -> VINP_ADASLDWSta_enum/1  "VINP_ADASLDWSta_enum"
  ADASLDWSta/2 -> Terminator_23/1
  [BHAL_outputs] -> slr_VHAL_ADASLFCHandsOffWarning_enum/1
  slr_VHAL_ADASLFCHandsOffWarning_enum/1 -> ADASLFCHandsOffWarning/1  "<VHAL_ADASLFCHandsOffWarning_enum>"
  True_VHAL_ADASLFCHandsOffWarning_enum/1 -> ADASLFCHandsOffWarning/2
  [inp_CanValid_bus] -> slr1_24/1
  slr1_24/1 -> ADASLFCHandsOffWarning/3  "<VINP_CANMsgValidFCM1_flg>"
  ADASLFCHandsOffWarning/1 -> VINP_ADASLFCHandsOffWarning_enum/1  "VINP_ADASLFCHandsOffWarning_enum"
  ADASLFCHandsOffWarning/2 -> Terminator_24/1
  [BHAL_outputs] -> slr_VHAL_ADASLFCSta_enum/1
  slr_VHAL_ADASLFCSta_enum/1 -> ADASLFCSta/1  "<VHAL_ADASLFCSta_enum>"
  True_VHAL_ADASLFCSta_enum/1 -> ADASLFCSta/2
  [inp_CanValid_bus] -> slr1_25/1
  slr1_25/1 -> ADASLFCSta/3  "<VINP_CANMsgValidFCM1_flg>"
  ADASLFCSta/1 -> VINP_ADASLFCSta_enum/1  "VINP_ADASLFCSta_enum"
  ADASLFCSta/2 -> Terminator_25/1
  [BHAL_outputs] -> slr_VHAL_ADASLFCWarnSound_enum/1
  slr_VHAL_ADASLFCWarnSound_enum/1 -> ADASLFCWarnSound/1  "<VHAL_ADASLFCWarnSound_enum>"
  True_VHAL_ADASLFCWarnSound_enum/1 -> ADASLFCWarnSound/2
  [inp_CanValid_bus] -> slr1_26/1
  slr1_26/1 -> ADASLFCWarnSound/3  "<VINP_CANMsgValidFCM1_flg>"
  ADASLFCWarnSound/1 -> VINP_ADASLFCWarnSound_enum/1  "VINP_ADASLFCWarnSound_enum"
  ADASLFCWarnSound/2 -> Terminator_26/1
  [BHAL_outputs] -> slr_VHAL_ADASLKASta_enum/1
  slr_VHAL_ADASLKASta_enum/1 -> ADASLKASta/1  "<VHAL_ADASLKASta_enum>"
  True_VHAL_ADASLKASta_enum/1 -> ADASLKASta/2
  [inp_CanValid_bus] -> slr1_27/1
  slr1_27/1 -> ADASLKASta/3  "<VINP_CANMsgValidFCM1_flg>"
  ADASLKASta/1 -> VINP_ADASLKASta_enum/1  "VINP_ADASLKASta_enum"
  ADASLKASta/2 -> Terminator_27/1
  [BHAL_outputs] -> slr_VHAL_ADASLaneModeL_enum/1
  slr_VHAL_ADASLaneModeL_enum/1 -> ADASLaneModeL/1  "<VHAL_ADASLaneModeL_enum>"
  True_VHAL_ADASLaneModeL_enum/1 -> ADASLaneModeL/2
  [inp_CanValid_bus] -> slr1_28/1
  slr1_28/1 -> ADASLaneModeL/3  "<VINP_CANMsgValidFCM1_flg>"
  ADASLaneModeL/1 -> VINP_ADASLaneModeL_enum/1  "VINP_ADASLaneModeL_enum"
  ADASLaneModeL/2 -> Terminator_28/1
  [BHAL_outputs] -> slr_VHAL_ADASLaneModeR_enum/1
  slr_VHAL_ADASLaneModeR_enum/1 -> ADASLaneModeR/1  "<VHAL_ADASLaneModeR_enum>"
  True_VHAL_ADASLaneModeR_enum/1 -> ADASLaneModeR/2
  [inp_CanValid_bus] -> slr1_29/1
  slr1_29/1 -> ADASLaneModeR/3  "<VINP_CANMsgValidFCM1_flg>"
  ADASLaneModeR/1 -> VINP_ADASLaneModeR_enum/1  "VINP_ADASLaneModeR_enum"
  ADASLaneModeR/2 -> Terminator_29/1
  [BHAL_outputs] -> slr_VHAL_ADASLanecurveL_raw32/1
  slr_VHAL_ADASLanecurveL_raw32/1 -> ADASLanecurveL/1  "<VHAL_ADASLanecurveL_raw32>"
  True_VHAL_ADASLanecurveL_raw32/1 -> ADASLanecurveL/2
  [inp_CanValid_bus] -> slr1_30/1
  slr1_30/1 -> ADASLanecurveL/3  "<VINP_CANMsgValidFCM1_flg>"
  ADASLanecurveL/1 -> VINP_ADASLanecurveL_raw32/1  "VINP_ADASLanecurveL_raw32"
  ADASLanecurveL/2 -> Terminator_30/1
  [BHAL_outputs] -> slr_VHAL_ADASLanecurveR_raw32/1
  slr_VHAL_ADASLanecurveR_raw32/1 -> ADASLanecurveR/1  "<VHAL_ADASLanecurveR_raw32>"
  True_VHAL_ADASLanecurveR_raw32/1 -> ADASLanecurveR/2
  [inp_CanValid_bus] -> slr1_31/1
  slr1_31/1 -> ADASLanecurveR/3  "<VINP_CANMsgValidFCM1_flg>"
  ADASLanecurveR/1 -> VINP_ADASLanecurveR_raw32/1  "VINP_ADASLanecurveR_raw32"
  ADASLanecurveR/2 -> Terminator_31/1
  [BHAL_outputs] -> slr_VHAL_ADASLanetypeL_enum/1
  slr_VHAL_ADASLanetypeL_enum/1 -> ADASLanetypeL/1  "<VHAL_ADASLanetypeL_enum>"
  True_VHAL_ADASLanetypeL_enum/1 -> ADASLanetypeL/2
  [inp_CanValid_bus] -> slr1_32/1
  slr1_32/1 -> ADASLanetypeL/3  "<VINP_CANMsgValidFCM1_flg>"
  ADASLanetypeL/1 -> VINP_ADASLanetypeL_enum/1  "VINP_ADASLanetypeL_enum"
  ADASLanetypeL/2 -> Terminator_32/1
  [BHAL_outputs] -> slr_VHAL_ADASLanetypeR_enum/1
  slr_VHAL_ADASLanetypeR_enum/1 -> ADASLanetypeR/1  "<VHAL_ADASLanetypeR_enum>"
  True_VHAL_ADASLanetypeR_enum/1 -> ADASLanetypeR/2
  [inp_CanValid_bus] -> slr1_33/1
  slr1_33/1 -> ADASLanetypeR/3  "<VINP_CANMsgValidFCM1_flg>"
  ADASLanetypeR/1 -> VINP_ADASLanetypeR_enum/1  "VINP_ADASLanetypeR_enum"
  ADASLanetypeR/2 -> Terminator_33/1
  [BHAL_outputs] -> slr_VHAL_ADASSLIFSpdLim_enum/1
  slr_VHAL_ADASSLIFSpdLim_enum/1 -> ADASSLIFSpdLim/1  "<VHAL_ADASSLIFSpdLim_enum>"
  True_VHAL_ADASSLIFSpdLim_enum/1 -> ADASSLIFSpdLim/2
  [inp_CanValid_bus] -> slr1_34/1
  slr1_34/1 -> ADASSLIFSpdLim/3  "<VINP_CANMsgValidFCM1_flg>"
  ADASSLIFSpdLim/1 -> VINP_ADASSLIFSpdLim_enum/1  "VINP_ADASSLIFSpdLim_enum"
  ADASSLIFSpdLim/2 -> Terminator_34/1
  [BHAL_outputs] -> slr_VHAL_ADASSLIFSta_enum/1
  slr_VHAL_ADASSLIFSta_enum/1 -> ADASSLIFSta/1  "<VHAL_ADASSLIFSta_enum>"
  True_VHAL_ADASSLIFSta_enum/1 -> ADASSLIFSta/2
  [inp_CanValid_bus] -> slr1_35/1
  slr1_35/1 -> ADASSLIFSta/3  "<VINP_CANMsgValidFCM1_flg>"
  ADASSLIFSta/1 -> VINP_ADASSLIFSta_enum/1  "VINP_ADASSLIFSta_enum"
  ADASSLIFSta/2 -> Terminator_35/1
  [BHAL_outputs] -> slr_VHAL_ADASShftPosnReq_enum/1
  slr_VHAL_ADASShftPosnReq_enum/1 -> ADASShftPosnReq/1  "<VHAL_ADASShftPosnReq_enum>"
  True_VHAL_ADASShftPosnReq_enum/1 -> ADASShftPosnReq/2
  [inp_CanValid_bus] -> slr1_36/1
  slr1_36/1 -> ADASShftPosnReq/3  "<VINP_CANMsgValidFCM1_flg>"
  ADASShftPosnReq/1 -> VINP_ADASShftPosnReq_enum/1  "VINP_ADASShftPosnReq_enum"
  ADASShftPosnReq/2 -> Terminator_36/1
  [BHAL_outputs] -> slr_VHAL_ADASShftPosnReqA_flg/1
  slr_VHAL_ADASShftPosnReqA_flg/1 -> ADASShftPosnReqA/1  "<VHAL_ADASShftPosnReqA_flg>"
  True_VHAL_ADASShftPosnReqA_flg/1 -> ADASShftPosnReqA/2
  [inp_CanValid_bus] -> slr1_37/1
  slr1_37/1 -> ADASShftPosnReqA/3  "<VINP_CANMsgValidFCM1_flg>"
  ADASShftPosnReqA/1 -> VINP_ADASShftPosnReqA_flg/1  "VINP_ADASShftPosnReqA_flg"
  ADASShftPosnReqA/2 -> Terminator_37/1
  [BHAL_outputs] -> slr_VHAL_ADASVehSpdLim_enum/1
  slr_VHAL_ADASVehSpdLim_enum/1 -> ADASVehSpdLim/1  "<VHAL_ADASVehSpdLim_enum>"
  True_VHAL_ADASVehSpdLim_enum/1 -> ADASVehSpdLim/2
  [inp_CanValid_bus] -> slr1_38/1
  slr1_38/1 -> ADASVehSpdLim/3  "<VINP_CANMsgValidFCM1_flg>"
  ADASVehSpdLim/1 -> VINP_ADASVehSpdLim_enum/1  "VINP_ADASVehSpdLim_enum"
  ADASVehSpdLim/2 -> Terminator_38/1
  [BHAL_outputs] -> slr_VHAL_ADASWarningMsg_enum/1
  slr_VHAL_ADASWarningMsg_enum/1 -> ADASWarningMsg/1  "<VHAL_ADASWarningMsg_enum>"
  True_VHAL_ADASWarningMsg_enum/1 -> ADASWarningMsg/2
  [inp_CanValid_bus] -> slr1_39/1
  slr1_39/1 -> ADASWarningMsg/3  "<VINP_CANMsgValidFCM1_flg>"
  ADASWarningMsg/1 -> VINP_ADASWarningMsg_enum/1  "VINP_ADASWarningMsg_enum"
  ADASWarningMsg/2 -> Terminator_39/1
  [BHAL_outputs] -> slr_VHAL_AEBVehHoldReq_flg/1
  slr_VHAL_AEBVehHoldReq_flg/1 -> AEBVehHoldReq/1  "<VHAL_AEBVehHoldReq_flg>"
  True_VHAL_AEBVehHoldReq_flg/1 -> AEBVehHoldReq/2
  [inp_CanValid_bus] -> slr1_40/1
  slr1_40/1 -> AEBVehHoldReq/3  "<VINP_CANMsgValidFCM1_flg>"
  AEBVehHoldReq/1 -> VINP_AEBVehHoldReq_flg/1  "VINP_AEBVehHoldReq_flg"
  AEBVehHoldReq/2 -> Terminator_40/1
  [BHAL_outputs] -> slr_VHAL_CameraBlockage_flg/1
  slr_VHAL_CameraBlockage_flg/1 -> CameraBlockage/1  "<VHAL_CameraBlockage_flg>"
  True_VHAL_CameraBlockage_flg/1 -> CameraBlockage/2
  [inp_CanValid_bus] -> slr1_41/1
  slr1_41/1 -> CameraBlockage/3  "<VINP_CANMsgValidFCM1_flg>"
  CameraBlockage/1 -> VINP_CameraBlockage_flg/1  "VINP_CameraBlockage_flg"
  CameraBlockage/2 -> Terminator_41/1
  [BHAL_outputs] -> slr_VHAL_FCM1Checksum_enum/1
  slr_VHAL_FCM1Checksum_enum/1 -> FCM1Checksum/1  "<VHAL_FCM1Checksum_enum>"
  True_VHAL_FCM1Checksum_enum/1 -> FCM1Checksum/2
  [inp_CanValid_bus] -> slr1_42/1
  slr1_42/1 -> FCM1Checksum/3  "<VINP_CANMsgValidFCM1_flg>"
  FCM1Checksum/1 -> VINP_FCM1Checksum_enum/1  "VINP_FCM1Checksum_enum"
  FCM1Checksum/2 -> Terminator_42/1
  [BHAL_outputs] -> slr_VHAL_FCM1LifeCount_enum/1
  slr_VHAL_FCM1LifeCount_enum/1 -> FCM1LifeCount/1  "<VHAL_FCM1LifeCount_enum>"
  True_VHAL_FCM1LifeCount_enum/1 -> FCM1LifeCount/2
  [inp_CanValid_bus] -> slr1_43/1
  slr1_43/1 -> FCM1LifeCount/3  "<VINP_CANMsgValidFCM1_flg>"
  FCM1LifeCount/1 -> VINP_FCM1LifeCount_enum/1  "VINP_FCM1LifeCount_enum"
  FCM1LifeCount/2 -> Terminator_43/1
  [BHAL_outputs] -> slr_VHAL_FCMACCmode_enum/1
  slr_VHAL_FCMACCmode_enum/1 -> FCMACCmode/1  "<VHAL_FCMACCmode_enum>"
  True_VHAL_FCMACCmode_enum/1 -> FCMACCmode/2
  [inp_CanValid_bus] -> slr1_44/1
  slr1_44/1 -> FCMACCmode/3  "<VINP_CANMsgValidFCM1_flg>"
  FCMACCmode/1 -> VINP_FCMACCmode_enum/1  "VINP_FCMACCmode_enum"
  FCMACCmode/2 -> Terminator_44/1
  [BHAL_outputs] -> slr_VHAL_FCMLKAStrToqReq_Nm/1
  slr_VHAL_FCMLKAStrToqReq_Nm/1 -> FCMLKAStrToqReq/1  "<VHAL_FCMLKAStrToqReq_Nm>"
  True_VHAL_FCMLKAStrToqReq_Nm/1 -> FCMLKAStrToqReq/2
  [inp_CanValid_bus] -> slr1_45/1
  slr1_45/1 -> FCMLKAStrToqReq/3  "<VINP_CANMsgValidFCM1_flg>"
  FCMLKAStrToqReq/1 -> VINP_FCMLKAStrToqReq_Nm/1  "VINP_FCMLKAStrToqReq_Nm"
  FCMLKAStrToqReq/2 -> Terminator_45/1
  [BHAL_outputs] -> slr_VHAL_FCMLKATOIAct_enum/1
  slr_VHAL_FCMLKATOIAct_enum/1 -> FCMLKATOIAct/1  "<VHAL_FCMLKATOIAct_enum>"
  True_VHAL_FCMLKATOIAct_enum/1 -> FCMLKATOIAct/2
  [inp_CanValid_bus] -> slr1_46/1
  slr1_46/1 -> FCMLKATOIAct/3  "<VINP_CANMsgValidFCM1_flg>"
  FCMLKATOIAct/1 -> VINP_FCMLKATOIAct_enum/1  "VINP_FCMLKATOIAct_enum"
  FCMLKATOIAct/2 -> Terminator_46/1
  [BHAL_outputs] -> slr_VHAL_FCMLKATOIFault_flg/1
  slr_VHAL_FCMLKATOIFault_flg/1 -> FCMLKATOIFault/1  "<VHAL_FCMLKATOIFault_flg>"
  True_VHAL_FCMLKATOIFault_flg/1 -> FCMLKATOIFault/2
  [inp_CanValid_bus] -> slr1_47/1
  slr1_47/1 -> FCMLKATOIFault/3  "<VINP_CANMsgValidFCM1_flg>"
  FCMLKATOIFault/1 -> VINP_FCMLKATOIFault_flg/1  "VINP_FCMLKATOIFault_flg"
  FCMLKATOIFault/2 -> Terminator_47/1
  [BHAL_outputs] -> slr_VHAL_ForceLowBeam_enum/1
  slr_VHAL_ForceLowBeam_enum/1 -> ForceLowBeam/1  "<VHAL_ForceLowBeam_enum>"
  True_VHAL_ForceLowBeam_enum/1 -> ForceLowBeam/2
  [inp_CanValid_bus] -> slr1_48/1
  slr1_48/1 -> ForceLowBeam/3  "<VINP_CANMsgValidFCM1_flg>"
  ForceLowBeam/1 -> VINP_ForceLowBeam_enum/1  "VINP_ForceLowBeam_enum"
  ForceLowBeam/2 -> Terminator_48/1
  [BHAL_outputs] -> slr_VHAL_HazardWarningReq_flg/1
  slr_VHAL_HazardWarningReq_flg/1 -> HazardWarningReq/1  "<VHAL_HazardWarningReq_flg>"
  True_VHAL_HazardWarningReq_flg/1 -> HazardWarningReq/2
  [inp_CanValid_bus] -> slr1_49/1
  slr1_49/1 -> HazardWarningReq/3  "<VINP_CANMsgValidFCM1_flg>"
  HazardWarningReq/1 -> VINP_HazardWarningReq_flg/1  "VINP_HazardWarningReq_flg"
  HazardWarningReq/2 -> Terminator_49/1
  [BHAL_outputs] -> slr_VHAL_ISAWarningMsg_enum/1
  slr_VHAL_ISAWarningMsg_enum/1 -> ISAWarningMsg/1  "<VHAL_ISAWarningMsg_enum>"
  True_VHAL_ISAWarningMsg_enum/1 -> ISAWarningMsg/2
  [inp_CanValid_bus] -> slr1_50/1
  slr1_50/1 -> ISAWarningMsg/3  "<VINP_CANMsgValidFCM1_flg>"
  ISAWarningMsg/1 -> VINP_ISAWarningMsg_enum/1  "VINP_ISAWarningMsg_enum"
  ISAWarningMsg/2 -> Terminator_50/1
  [BHAL_outputs] -> slr_VHAL_LKAHODDisplayWarning_flg/1
  slr_VHAL_LKAHODDisplayWarning_flg/1 -> LKAHODDisplayWarning/1  "<VHAL_LKAHODDisplayWarning_flg>"
  True_VHAL_LKAHODDisplayWarning_flg/1 -> LKAHODDisplayWarning/2
  [inp_CanValid_bus] -> slr1_51/1
  slr1_51/1 -> LKAHODDisplayWarning/3  "<VINP_CANMsgValidFCM1_flg>"
  LKAHODDisplayWarning/1 -> VINP_LKAHODDisplayWarning_flg/1  "VINP_LKAHODDisplayWarning_flg"
  LKAHODDisplayWarning/2 -> Terminator_51/1
  [BHAL_outputs] -> slr_VHAL_LKAHODSoundWarning_flg/1
  slr_VHAL_LKAHODSoundWarning_flg/1 -> LKAHODSoundWarning/1  "<VHAL_LKAHODSoundWarning_flg>"
  True_VHAL_LKAHODSoundWarning_flg/1 -> LKAHODSoundWarning/2
  [inp_CanValid_bus] -> slr1_52/1
  slr1_52/1 -> LKAHODSoundWarning/3  "<VINP_CANMsgValidFCM1_flg>"
  LKAHODSoundWarning/1 -> VINP_LKAHODSoundWarning_flg/1  "VINP_LKAHODSoundWarning_flg"
  LKAHODSoundWarning/2 -> Terminator_52/1
  [BHAL_outputs] -> slr_VHAL_LVDAACCStatusInformation_flg/1
  slr_VHAL_LVDAACCStatusInformation_flg/1 -> LVDAACCStatusInformation/1  "<VHAL_LVDAACCStatusInformation_flg>"
  True_VHAL_LVDAACCStatusInformation_flg/1 -> LVDAACCStatusInformation/2
  [inp_CanValid_bus] -> slr1_53/1
  slr1_53/1 -> LVDAACCStatusInformation/3  "<VINP_CANMsgValidFCM1_flg>"
  LVDAACCStatusInformation/1 -> VINP_LVDAACCStatusInformation_flg/1  "VINP_LVDAACCStatusInformation_flg"
  LVDAACCStatusInformation/2 -> Terminator_53/1
  [BHAL_outputs] -> slr_VHAL_LVDADisabled_flg/1
  slr_VHAL_LVDADisabled_flg/1 -> LVDADisabled/1  "<VHAL_LVDADisabled_flg>"
  True_VHAL_LVDADisabled_flg/1 -> LVDADisabled/2
  [inp_CanValid_bus] -> slr1_54/1
  slr1_54/1 -> LVDADisabled/3  "<VINP_CANMsgValidFCM1_flg>"
  LVDADisabled/1 -> VINP_LVDADisabled_flg/1  "VINP_LVDADisabled_flg"
  LVDADisabled/2 -> Terminator_54/1
  [BHAL_outputs] -> slr_VHAL_LVDAFailinfo_flg/1
  slr_VHAL_LVDAFailinfo_flg/1 -> LVDAFailinfo/1  "<VHAL_LVDAFailinfo_flg>"
  True_VHAL_LVDAFailinfo_flg/1 -> LVDAFailinfo/2
  [inp_CanValid_bus] -> slr1_55/1
  slr1_55/1 -> LVDAFailinfo/3  "<VINP_CANMsgValidFCM1_flg>"
  LVDAFailinfo/1 -> VINP_LVDAFailinfo_flg/1  "VINP_LVDAFailinfo_flg"
  LVDAFailinfo/2 -> Terminator_55/1
  [BHAL_outputs] -> slr_VHAL_LVDAMuteSta_enum/1
  slr_VHAL_LVDAMuteSta_enum/1 -> LVDAMuteSta/1  "<VHAL_LVDAMuteSta_enum>"
  True_VHAL_LVDAMuteSta_enum/1 -> LVDAMuteSta/2
  [inp_CanValid_bus] -> slr1_56/1
  slr1_56/1 -> LVDAMuteSta/3  "<VINP_CANMsgValidFCM1_flg>"
  LVDAMuteSta/1 -> VINP_LVDAMuteSta_enum/1  "VINP_LVDAMuteSta_enum"
  LVDAMuteSta/2 -> Terminator_56/1
  [BHAL_outputs] -> slr_VHAL_LVDAWarning_flg/1
  slr_VHAL_LVDAWarning_flg/1 -> LVDAWarning/1  "<VHAL_LVDAWarning_flg>"
  True_VHAL_LVDAWarning_flg/1 -> LVDAWarning/2
  [inp_CanValid_bus] -> slr1_57/1
  slr1_57/1 -> LVDAWarning/3  "<VINP_CANMsgValidFCM1_flg>"
  LVDAWarning/1 -> VINP_LVDAWarning_flg/1  "VINP_LVDAWarning_flg"
  LVDAWarning/2 -> Terminator_57/1
  [BHAL_outputs] -> slr_VHAL_LeftTurnLightReq_flg/1
  slr_VHAL_LeftTurnLightReq_flg/1 -> LeftTurnLightReq/1  "<VHAL_LeftTurnLightReq_flg>"
  True_VHAL_LeftTurnLightReq_flg/1 -> LeftTurnLightReq/2
  [inp_CanValid_bus] -> slr1_58/1
  slr1_58/1 -> LeftTurnLightReq/3  "<VINP_CANMsgValidFCM1_flg>"
  LeftTurnLightReq/1 -> VINP_LeftTurnLightReq_flg/1  "VINP_LeftTurnLightReq_flg"
  LeftTurnLightReq/2 -> Terminator_58/1
  [BHAL_outputs] -> slr_VHAL_RightTurnLightReq_flg/1
  slr_VHAL_RightTurnLightReq_flg/1 -> RightTurnLightReq/1  "<VHAL_RightTurnLightReq_flg>"
  True_VHAL_RightTurnLightReq_flg/1 -> RightTurnLightReq/2
  [inp_CanValid_bus] -> slr1_59/1
  slr1_59/1 -> RightTurnLightReq/3  "<VINP_CANMsgValidFCM1_flg>"
  RightTurnLightReq/1 -> VINP_RightTurnLightReq_flg/1  "VINP_RightTurnLightReq_flg"
  RightTurnLightReq/2 -> Terminator_59/1
  [BHAL_outputs] -> slr_VHAL_TargetType_enum/1
  slr_VHAL_TargetType_enum/1 -> TargetType/1  "<VHAL_TargetType_enum>"
  True_VHAL_TargetType_enum/1 -> TargetType/2
  [inp_CanValid_bus] -> slr1_60/1
  slr1_60/1 -> TargetType/3  "<VINP_CANMsgValidFCM1_flg>"
  TargetType/1 -> VINP_TargetType_enum/1  "VINP_TargetType_enum"
  TargetType/2 -> Terminator_60/1
  [BHAL_outputs] -> slr_VHAL_TimeGapLevel_enum/1
  slr_VHAL_TimeGapLevel_enum/1 -> TimeGapLevel/1  "<VHAL_TimeGapLevel_enum>"
  True_VHAL_TimeGapLevel_enum/1 -> TimeGapLevel/2
  [inp_CanValid_bus] -> slr1_61/1
  slr1_61/1 -> TimeGapLevel/3  "<VINP_CANMsgValidFCM1_flg>"
  TimeGapLevel/1 -> VINP_TimeGapLevel_enum/1  "VINP_TimeGapLevel_enum"
  TimeGapLevel/2 -> Terminator_61/1
